simulink model "actual_model_v2"  (R2022a)
settings: Solver=ode23t  StartTime=0.0  StopTime=10  FixedStep=0.001  RelTol=1e-3
undefined symbols (not defined in the file or in its folder): A, B, C, C_lqr, Const_input, D, Kr, x_des
settings Model: Creator=asmax  LastModifiedBy=asmax
settings SolverCC: EnableFixedStepZeroCrossing=on

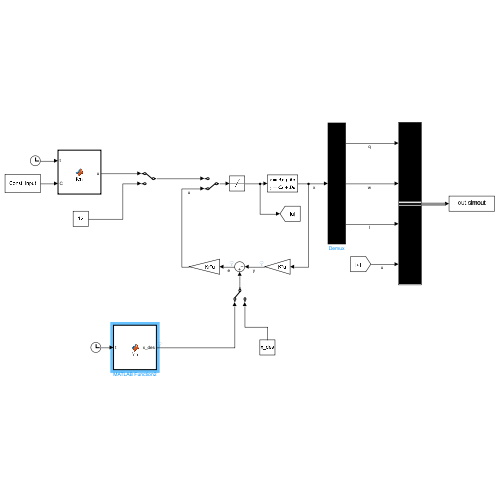
[thumbnail: Simulink's stored preview of the top-level diagram]
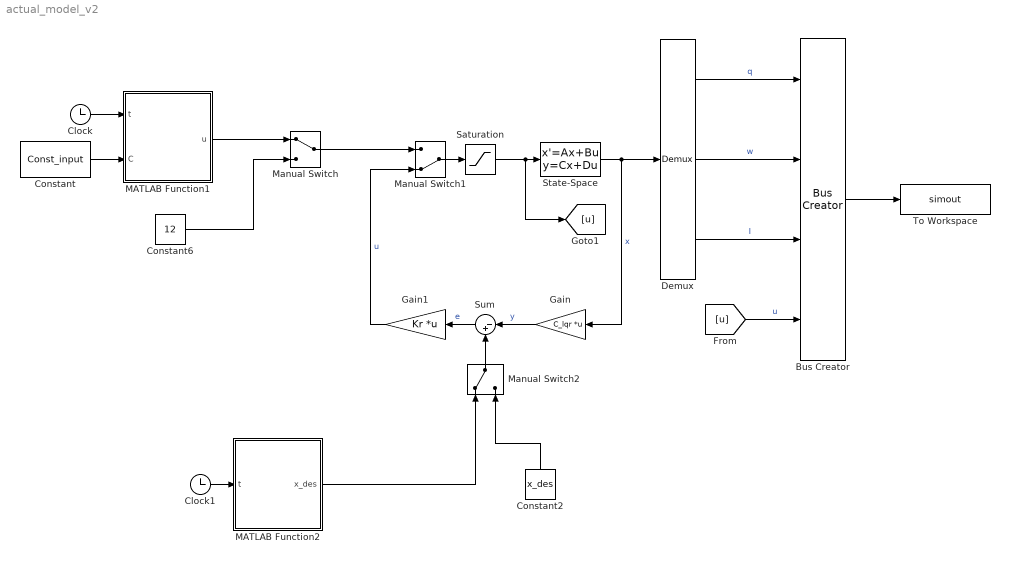
== system actual_model_v2 ==
  Bus Creator : BusCreator  Inputs=4
  Clock : Clock
  Clock1 : Clock
  Constant : Constant  Value=Const_input
  Constant2 : Constant  Value=x_des
  Constant6 : Constant  Value=12
  Demux : Demux  Outputs=3
  Gain : Gain  Gain=C_lqr  Multiplication=Matrix(K*u)
  Gain1 : Gain  Gain=Kr  Multiplication=Matrix(K*u)
  MATLAB Function1 : MATLAB Function  TreatAsAtomicUnit=on
  MATLAB Function2 : MATLAB Function  TreatAsAtomicUnit=on
  Manual Switch : ManualSwitch
  Manual Switch1 : ManualSwitch  CurrentSetting=0
  Manual Switch2 : ManualSwitch
  Saturation : Saturate  UpperLimit=15  LowerLimit=-15
  State-Space : StateSpace  A=A  B=B  C=C  D=D  InitialCondition=[0 0 0]'
  Sum : Sum  Inputs=|-+
  To Workspace : ToWorkspace  VariableName=simout  SaveFormat=Timeseries  SampleTime=-1
  wires:
  Clock/1 -> MATLAB Function1/1(t)
  MATLAB Function1/1(u) -> Manual Switch/1
  Constant6/1 -> Manual Switch/2
  Constant/1 -> MATLAB Function1/2(C)
  State-Space/1 -> Gain/1, Demux/1  "x"
  Bus Creator/1 -> To Workspace/1
  Demux/2 -> Bus Creator/2  "w"
  Demux/1 -> Bus Creator/1  "q"
  [u] -> Bus Creator/4  "u"
  Gain/1 -> Sum/1  "y"
  Manual Switch1/1 -> Saturation/1
  Gain1/1 -> Manual Switch1/2  "u"
  Manual Switch/1 -> Manual Switch1/1
  Sum/1 -> Gain1/1  "e"
  Demux/3 -> Bus Creator/3  "I"
  Clock1/1 -> MATLAB Function2/1(t)
  Manual Switch2/1 -> Sum/2
  Constant2/1 -> Manual Switch2/2
  MATLAB Function2/1(x_des) -> Manual Switch2/1
  Saturation/1 -> [u], State-Space/1

== matlab function actual_model_v2/MATLAB Function1 ==
  data: t input; u output; C input
function u = fcn(t, C)

% w = 4;
% A = 6;
% B = 6;
% fi = 3.1415;
% u = A * cos(w * t + fi) + B;

w = C(3);
A = C(1);
B = C(2);
fi = C(4);
u = A * cos(w * t + fi) + B;

== matlab function actual_model_v2/MATLAB Function2 ==
  data: t input; x_des output
function x_des = fcn(t)

w = 2;
A = 400;
B = A;
fi = 3.1415;
% w_des = A * cos(w * t + fi) + B;
w_des = -A*w * sin(w * t + fi);

w = 2;
A = 400;
B = A;
fi = 3.1415;
q_des = A * cos(w * t + fi) + B;

% x_des = [0 w_des 0]';
% x_des = [q_des 0 0]';
x_des = [q_des w_des 0]';
